simulink model "RB_Simulation"  (R2017b)
settings: Solver=VariableStepAuto  StartTime=0.0  StopTime=10.0  FixedStep=0.01  MaxStep=0.01  RelTol=1e-3
settings Model: Creator=guoro  LastModifiedBy=guoro

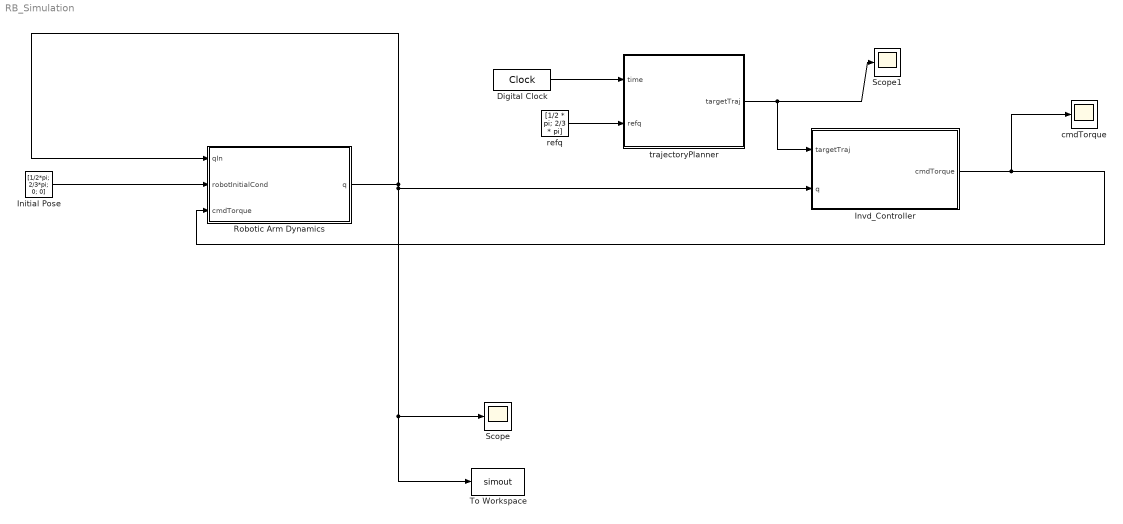
== system RB_Simulation ==
  Digital Clock : DigitalClock
  Initial Pose : Constant  Value=[1/2*pi; 2/3*pi; 0; 0]  VectorParams1D=off
  "Invd_Controller " : Subsystem
      mask Display: image('C:\Users\guoro\Downloads\WeChat Image_20220811225038.jpg');
  Robotic Arm Dynamics : Subsystem
      mask Display: image('C:\Users\guoro\Downloads\WeChat Image_20220811224032.jpg');
  Scope : Scope
  Scope1 : Scope
  To Workspace : ToWorkspace  VariableName=simout  SaveFormat=Timeseries  SampleTime=-1
  cmdTorque : Scope
  refq : Constant  Value=[1/2 * pi; 2/3 * pi]
  trajectoryPlanner : MATLAB Function  TreatAsAtomicUnit=on
  wires:
  Robotic Arm Dynamics/1(q) -> To Workspace/1, Scope/1, "Invd_Controller "/2(q), Robotic Arm Dynamics/1(qIn)
  Initial Pose/1 -> Robotic Arm Dynamics/2(robotInitialCond)
  "Invd_Controller "/1(cmdTorque) -> cmdTorque/1, Robotic Arm Dynamics/3(cmdTorque)
  refq/1 -> trajectoryPlanner/2(refq)
  Digital Clock/1 -> trajectoryPlanner/1(time)
  trajectoryPlanner/1(targetTraj) -> Scope1/1, "Invd_Controller "/1("targetTraj ")

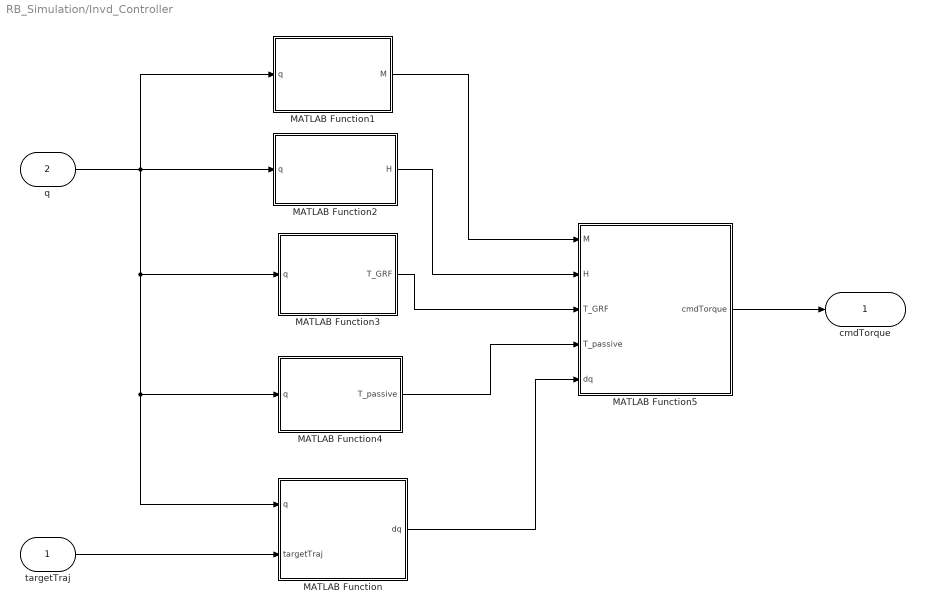
== system RB_Simulation/Invd_Controller  ==
  "targetTraj " : Inport
  q : Inport  Port=2
  MATLAB Function : MATLAB Function  TreatAsAtomicUnit=on
  MATLAB Function1 : MATLAB Function  TreatAsAtomicUnit=on
  MATLAB Function2 : MATLAB Function  TreatAsAtomicUnit=on
  MATLAB Function3 : MATLAB Function  TreatAsAtomicUnit=on
  MATLAB Function4 : MATLAB Function  TreatAsAtomicUnit=on
  MATLAB Function5 : MATLAB Function  TreatAsAtomicUnit=on
  cmdTorque : Outport
  wires:
  q/1 -> MATLAB Function/1(q), MATLAB Function4/1(q), MATLAB Function3/1(q), MATLAB Function1/1(q), MATLAB Function2/1(q)
  "targetTraj "/1 -> MATLAB Function/2(targetTraj)
  MATLAB Function1/1(M) -> MATLAB Function5/1(M)
  MATLAB Function2/1(H) -> MATLAB Function5/2(H)
  MATLAB Function3/1(T_GRF) -> MATLAB Function5/3(T_GRF)
  MATLAB Function4/1(T_passive) -> MATLAB Function5/4(T_passive)
  MATLAB Function/1(dq) -> MATLAB Function5/5(dq)
  MATLAB Function5/1(cmdTorque) -> cmdTorque/1

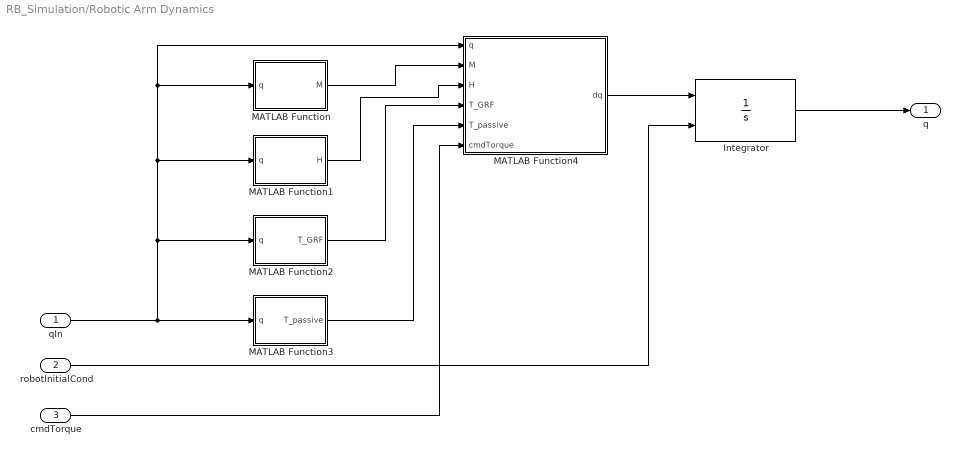
== system RB_Simulation/Robotic Arm Dynamics ==
  qIn : Inport
  robotInitialCond : Inport  Port=2
  cmdTorque : Inport  Port=3
  Integrator : Integrator  InitialConditionSource=external  InitialCondition=[1/2 * pi; 2/3 * pi; 0; 0]
  MATLAB Function : MATLAB Function  TreatAsAtomicUnit=on
  MATLAB Function1 : MATLAB Function  TreatAsAtomicUnit=on
  MATLAB Function2 : MATLAB Function  TreatAsAtomicUnit=on
  MATLAB Function3 : MATLAB Function  TreatAsAtomicUnit=on
  MATLAB Function4 : MATLAB Function  TreatAsAtomicUnit=on
  q : Outport
  wires:
  MATLAB Function/1(M) -> MATLAB Function4/2(M)
  cmdTorque/1 -> MATLAB Function4/6(cmdTorque)
  MATLAB Function3/1(T_passive) -> MATLAB Function4/5(T_passive)
  MATLAB Function1/1(H) -> MATLAB Function4/3(H)
  Integrator/1 -> q/1
  qIn/1 -> MATLAB Function1/1(q), MATLAB Function4/1(q), MATLAB Function/1(q), MATLAB Function2/1(q), MATLAB Function3/1(q)
  MATLAB Function4/1(dq) -> Integrator/1
  MATLAB Function2/1(T_GRF) -> MATLAB Function4/4(T_GRF)
  robotInitialCond/1 -> Integrator/2

== matlab function RB_Simulation/Robotic Arm Dynamics/MATLAB Function1 ==
  data: q input; H output
function H = coriolisTerm(q)
    H = [49.05  * cos(q(1)) - 6.13125 * cos(q(1)) * cos(q(2)) + 6.13125 * sin(q(1)) * sin(q(2)) + 0.625 * sin(q(2)) * q(3) * q(4) + 0.3125 * sin(q(2)) * q(4)^2;
         -6.13125 * cos(q(1)) * cos(q(2)) + 6.13125 * sin(q(1)) * sin(q(2)) - 0.3125 * sin(q(2)) * q(3)^2];
end

== matlab function RB_Simulation/Robotic Arm Dynamics/MATLAB Function ==
  data: q input; M output
function M = massMatrix(q)
 %% Lagrange-Euler Method : Mass Matrix
 M = [2.1875 - 0.625 * cos(q(2)), 0.104167 - 0.3125 * cos(q(2)); 0.104167 - 0.3125 * cos(q(2)), 0.104167];
end

== matlab function RB_Simulation/Robotic Arm Dynamics/MATLAB Function2 ==
  data: q input; T_GRF output
function T_GRF = groundRForce(q)
    T_GRF = [0; 0];
end

== matlab function RB_Simulation/Robotic Arm Dynamics/MATLAB Function3 ==
  data: q input; T_passive output
function T_passive = passiveJoint(q)
    % Passive Joint Constants
    Ks1 = 70;
    Bs1 = 5;
    Ks2 = 30;
    Bs2 = 5;
    theta_eq1 = 2/3 * pi;
    theta_eq2 = 1/2 * pi;
    % Passive Torque Calculation
    T_passive = [-Ks1 * (q(1) - theta_eq1) - Bs1 * q(3); -Ks2 * (q(2) - theta_eq2) - Bs2 * (q(4))];
end

== matlab function RB_Simulation/Robotic Arm Dynamics/MATLAB Function4 ==
  data: q input; dq output; M input; H input; T_GRF input; T_passive input; cmdTorque input
function dq = InverseDynamics(q, M, H, T_GRF, T_passive, cmdTorque)
    dq = zeros(4, 1);
    dq(1:2) = q(3:4);
    % Forward Kinematics
    k = -H + T_GRF + T_passive + cmdTorque;
    dq(3) = (M(1, 2) * k(2) - M(2, 2) * k(1)) / (M(1, 2) * M(2, 1) - M(1, 1) * M(2, 2));
    dq(4) = - (M(1, 1) * k(2) - M(2, 1) * k(1)) / (M(1, 2) * M(2, 1) - M(1, 1) * M(2, 2));
end

== matlab function RB_Simulation/Invd_Controller /MATLAB Function ==
  data: q input; dq output; targetTraj input
function dq = planner(q, targetTraj)
    Kp = 120;
    Kd = 15;
    dq = Kp * (targetTraj - q(1:2)) - Kd * q(3:4);
end

== matlab function RB_Simulation/Invd_Controller /MATLAB Function1 ==
  data: q input; M output
function M = massMatrix(q)
 %% Lagrange-Euler Method : Mass Matrix
 M = [2.1875 - 0.625 * cos(q(2)), 0.104167 - 0.3125 * cos(q(2)); 0.104167 - 0.3125 * cos(q(2)), 0.104167];
end

== matlab function RB_Simulation/Invd_Controller /MATLAB Function2 ==
  data: q input; H output
function H = coriolisTerm(q)
    H = [49.05  * cos(q(1)) - 6.13125 * cos(q(1)) * cos(q(2)) + 6.13125 * sin(q(1)) * sin(q(2)) + 0.625 * sin(q(2)) * q(3) * q(4) + 0.3125 * sin(q(2)) * q(4)^2;
         -6.13125 * cos(q(1)) * cos(q(2)) + 6.13125 * sin(q(1)) * sin(q(2)) - 0.3125 * sin(q(2)) * q(3)^2];
end

== matlab function RB_Simulation/Invd_Controller /MATLAB Function3 ==
  data: q input; T_GRF output
function T_GRF = groundRForce(q)
    T_GRF = [0; 0];
end

== matlab function RB_Simulation/Invd_Controller /MATLAB Function4 ==
  data: q input; T_passive output
function T_passive = passiveJoint(q)
    % Passive Joint Constants
    Ks1 = 70;
    Bs1 = 5;
    Ks2 = 30;
    Bs2 = 5;
    theta_eq1 = 2/3 * pi;
    theta_eq2 = 1/2 * pi;
    % Passive Torque Calculation
    T_passive = [-Ks1 * (q(1) - theta_eq1) - Bs1 * q(3); -Ks2 * (q(2) - theta_eq2) - Bs2 * (q(4))];
end

== matlab function RB_Simulation/Invd_Controller /MATLAB Function5 ==
  data: M input; cmdTorque output; H input; T_GRF input; T_passive input; dq input
function cmdTorque = InverseDynamics(M, H, T_GRF, T_passive, dq)
    cmdTorque = M * dq + H - T_passive - T_GRF;
end

== matlab function RB_Simulation/trajectoryPlanner ==
  data: time input; targetTraj output; refq input
function targetTraj = timeBased(time, refq)
    if (time >= 0 && time < 5)
        targetTraj = 0.7 * refq;
    elseif (time >= 5 && time < 8)
        targetTraj = 1 * refq;
    else
        targetTraj = 1.2 * refq;
    end
end
